simulink model "ADRC_SIMU_Blocks"  (R2018b)
settings: Solver=VariableStepAuto  StartTime=0.0  StopTime=10.0  RelTol=1e-3
settings Model: Creator=Whtest  LastModifiedBy=Whtest

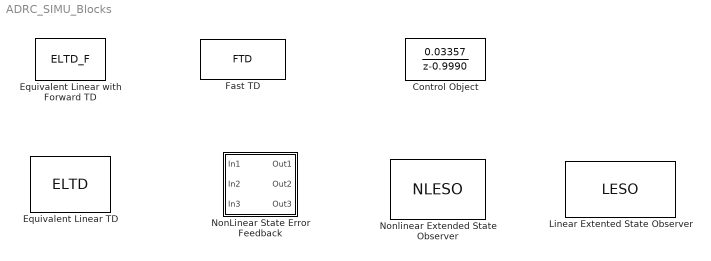
== system ADRC_SIMU_Blocks ==
  Control Object : DiscreteTransferFcn  Numerator="[0    0.03357]"  Denominator="[ 1.0000   -0.9990]"
  Equivalent Linear TD : S-Function  FunctionName=ELTD  Parameters=1,2,4  SFunctionDeploymentMode=off  EnableBusSupport=off
  Equivalent Linear with Forward TD : S-Function  FunctionName=ELTD_F  Parameters=1,1,2,3  SFunctionDeploymentMode=off  EnableBusSupport=off
  Fast TD : S-Function  FunctionName=FTD  Parameters=1E-3,1E-2,1000  SFunctionDeploymentMode=off  EnableBusSupport=off
  Linear Extented State Observer : S-Function  FunctionName=LESO  SFunctionDeploymentMode=off  EnableBusSupport=off
  NonLinear State Error Feedback : Subsystem
  Nonlinear Extended State Observer : S-Function  FunctionName=NLESO  Parameters=0.1,0.5,10,100,500,50  SFunctionDeploymentMode=off  EnableBusSupport=off

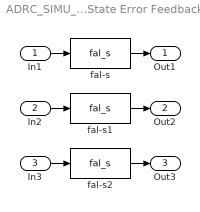
== system ADRC_SIMU_Blocks/NonLinear State Error Feedback ==
  In1 : Inport
  In2 : Inport  Port=2
  In3 : Inport  Port=3
  fal-s : S-Function  FunctionName=fal_s  Parameters=.5,0.5  SFunctionDeploymentMode=off  EnableBusSupport=off
  fal-s1 : S-Function  FunctionName=fal_s  Parameters=.5,0.5  SFunctionDeploymentMode=off  EnableBusSupport=off
  fal-s2 : S-Function  FunctionName=fal_s  Parameters=.5,0.5  SFunctionDeploymentMode=off  EnableBusSupport=off
  Out1 : Outport
  Out2 : Outport  Port=2
  Out3 : Outport  Port=3
  wires:
  In1/1 -> fal-s/1
  fal-s2/1 -> Out3/1
  In2/1 -> fal-s1/1
  fal-s1/1 -> Out2/1
  fal-s/1 -> Out1/1
  In3/1 -> fal-s2/1
